simulink model "Project1_Part2_Op2"  (R2023b)
settings: Solver=ode45  StartTime=0.0  StopTime=25  FixedStep=1  RelTol=1e-3
values from neighbouring files (symbols this model uses):
  b1 = 1    [Project1_Part2.m]
  b2 = 1    [Project1_Part2.m]
  const_torque = 1    [Project1_Part2.m]
  J1 = 100    [Project1_Part2.m]
  J2 = 1    [Project1_Part2.m]
settings Model: Creator=flare  LastModifiedBy=flare
settings DataIOCC: ReturnWorkspaceOutputsName=out2

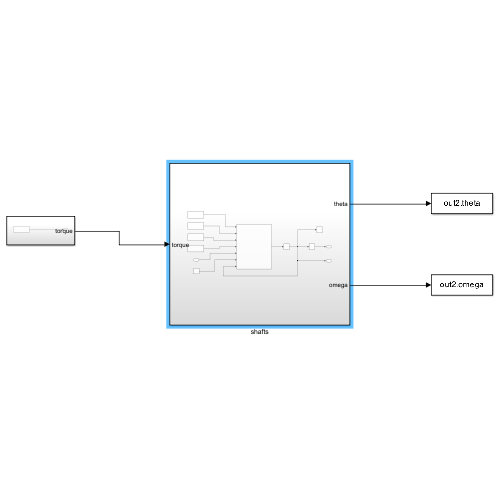
[thumbnail: Simulink's stored preview of the top-level diagram]
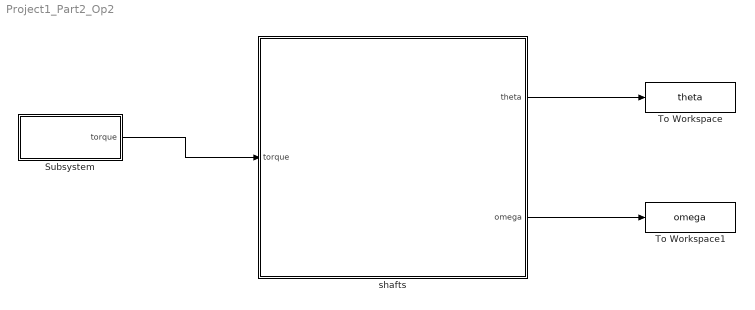
== system Project1_Part2_Op2 ==
  Subsystem : Subsystem
  To Workspace : ToWorkspace  VariableName=theta  SaveFormat=Timeseries  SampleTime=-1
  To Workspace1 : ToWorkspace  VariableName=omega  SaveFormat=Timeseries  SampleTime=-1
  shafts : Subsystem
  wires:
  Subsystem/1(torque) -> shafts/1(torque)
  shafts/1(theta) -> To Workspace/1
  shafts/2(omega) -> To Workspace1/1

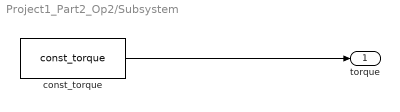
== system Project1_Part2_Op2/Subsystem ==
  const_torque : Constant  Value=const_torque
  torque : Outport
  wires:
  const_torque/1 -> torque/1

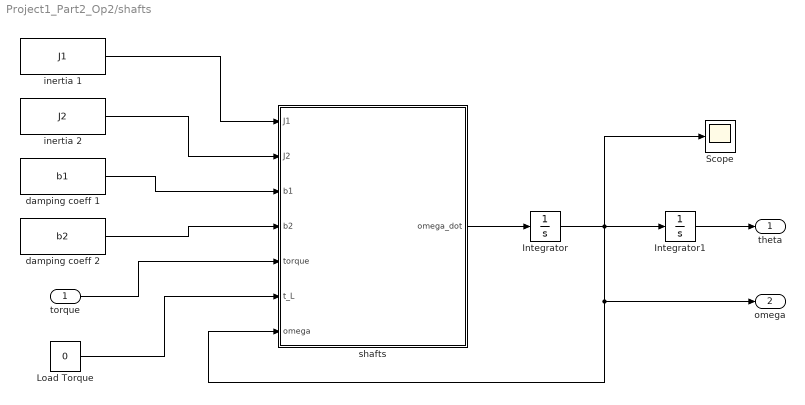
== system Project1_Part2_Op2/shafts ==
  torque : Inport
  Integrator : Integrator
  Integrator1 : Integrator
  Load Torque : Constant  Value=0
  Scope : Scope
  damping coeff 1 : Constant  Value=b1
  damping coeff 2 : Constant  Value=b2
  inertia 1 : Constant  Value=J1
  inertia 2 : Constant  Value=J2
  shafts : MATLAB Function  TreatAsAtomicUnit=on
  theta : Outport
  omega : Outport  Port=2
  wires:
  inertia 1/1 -> shafts/1(J1)
  inertia 2/1 -> shafts/2(J2)
  damping coeff 1/1 -> shafts/3(b1)
  damping coeff 2/1 -> shafts/4(b2)
  torque/1 -> shafts/5(torque)
  Load Torque/1 -> shafts/6(t_L)
  shafts/1(omega_dot) -> Integrator/1
  Integrator/1 -> Scope/1, omega/1, shafts/7(omega), Integrator1/1
  Integrator1/1 -> theta/1

== matlab function Project1_Part2_Op2/shafts/shafts ==
  data: J1 input; omega_dot output; J2 input; b1 input; b2 input; torque input; t_L input; omega input
function omega_dot = fcn(J1, J2, b1, b2, torque, t_L, omega)

J_c = J1 + J2;
b_c = b1 + b2;

omega_dot = (1/J_c)*(torque-t_L)-((b_c/J_c)*omega);
